simulink model "Robot 2"  (R2019a)
settings: Solver=VariableStepAuto  StartTime=0.0  StopTime=10.0  RelTol=1e-3
undefined symbols (not defined in the file): DiscIntNeverNeededParam
settings Model: Creator=mrblissfulgrin  LastModifiedBy=mrblissfulgrin

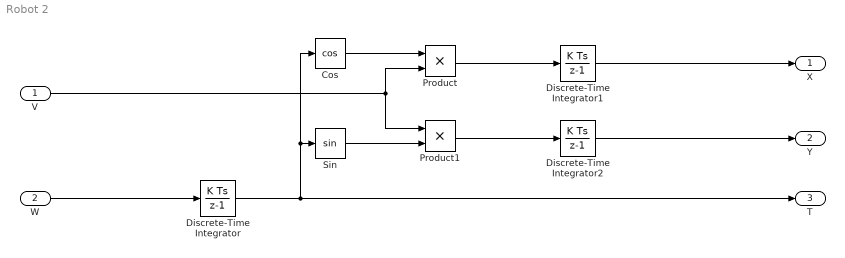
== system Robot 2 ==
  V : Inport
  W : Inport  Port=2
  Cos : Trigonometry  Operator=cos
  Discrete-Time Integrator : DiscreteIntegrator  InitialCondition=30*pi/180  SampleTime=0.01  ICPrevOutput=DiscIntNeverNeededParam  ICPrevScaledInput=DiscIntNeverNeededParam
  Discrete-Time Integrator1 : DiscreteIntegrator  SampleTime=0.01  ICPrevOutput=DiscIntNeverNeededParam  ICPrevScaledInput=DiscIntNeverNeededParam
  Discrete-Time Integrator2 : DiscreteIntegrator  SampleTime=0.01  ICPrevOutput=DiscIntNeverNeededParam  ICPrevScaledInput=DiscIntNeverNeededParam
  Product : Product
  Product1 : Product
  Sin : Trigonometry
  X : Outport
  Y : Outport  Port=2
  T : Outport  Port=3
  wires:
  W/1 -> Discrete-Time Integrator/1
  Discrete-Time Integrator/1 -> Sin/1, Cos/1, T/1
  Sin/1 -> Product1/2
  V/1 -> Product/2, Product1/1
  Product1/1 -> Discrete-Time Integrator2/1
  Product/1 -> Discrete-Time Integrator1/1
  Discrete-Time Integrator2/1 -> Y/1
  Discrete-Time Integrator1/1 -> X/1
  Cos/1 -> Product/1
